simulink model "sen_gyro_test"  (R2020b)
settings: Solver=FixedStepDiscrete  StartTime=0.0  StopTime=0  FixedStep=sen.imu_rate  RelTol=1e-3
undefined symbols (not defined in the file or in its folder): sen
settings Model: Creator=jsint  LastModifiedBy=jsint

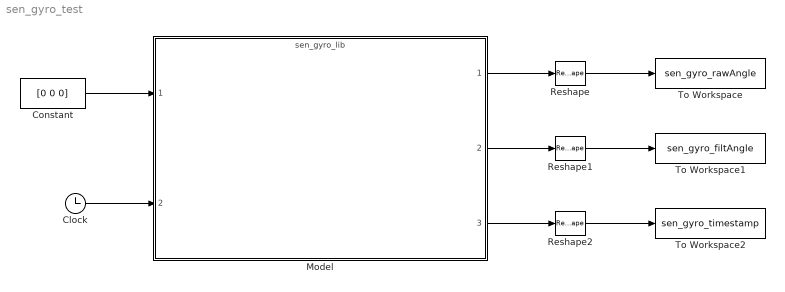
== system sen_gyro_test ==
  Clock : Clock
  Constant : Constant  Value=[0 0 0]
  Model : ModelReference  ModelNameDialog=sen_gyro_lib.slx  SimulationMode=Normal  ModelReferenceVersion=1.140
  Reshape : Reshape
  Reshape1 : Reshape
  Reshape2 : Reshape
  To Workspace : ToWorkspace  VariableName=sen_gyro_rawAngle  SaveFormat=Timeseries  SampleTime=sen.imu_rate
  To Workspace1 : ToWorkspace  VariableName=sen_gyro_filtAngle  SaveFormat=Timeseries  SampleTime=sen.imu_rate
  To Workspace2 : ToWorkspace  VariableName=sen_gyro_timestamp  SaveFormat=Timeseries  SampleTime=sen.imu_rate
  wires:
  Clock/1 -> Model/2
  Constant/1 -> Model/1
  Model/2 -> Reshape1/1
  Model/3 -> Reshape2/1
  Model/1 -> Reshape/1
  Reshape/1 -> To Workspace/1
  Reshape1/1 -> To Workspace1/1
  Reshape2/1 -> To Workspace2/1
